simulink model "Problem1"  (R2020b)
settings: Solver=VariableStepAuto  StartTime=0.0  StopTime=100  MaxStep=0.01  RelTol=1e-3
model workspace (MAT data in the model file):
  K12 = 5000
  M2 = 50
undefined symbols (not defined in the file): b, K1, M1
settings Model: Creator=Hp  LastModifiedBy=Makrand Raut Dessai

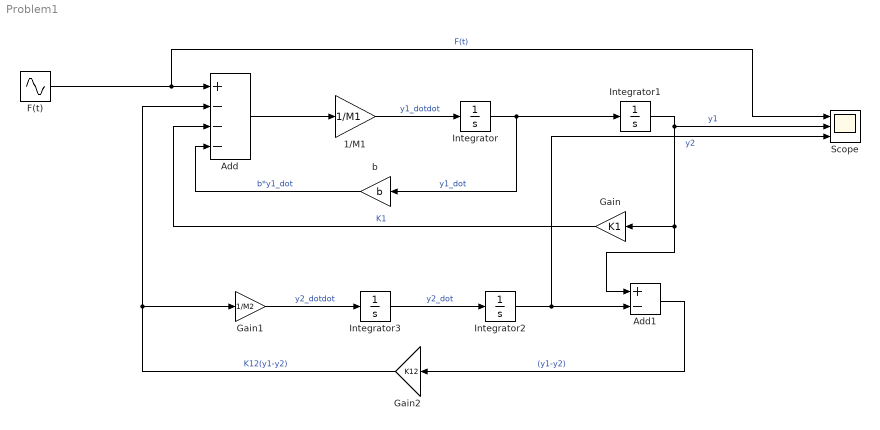
== system Problem1 ==
  1/M1 : Gain  Gain=1/M1
  Add : Sum  Inputs=+---
  Add1 : Sum  Inputs=+-
  F(t) : Sin  Amplitude=2  Frequency=10  SampleTime=0
  Gain : Gain  Gain=K1
  Gain1 : Gain  Gain=1/M2
  Gain2 : Gain  Gain=K12
  Integrator{,1..3} (4 alike) : Integrator
  Scope : Scope  NumInputPorts=3
  b : Gain  Gain=b
  wires:
  Gain2/1 -> Gain1/1, Add/2  "K12(y1-y2)"
  Add1/1 -> Gain2/1  "(y1-y2)"
  Integrator3/1 -> Integrator2/1  "y2_dot"
  1/M1/1 -> Integrator/1  "y1_dotdot"
  Integrator1/1 -> Scope/2, Gain/1, Add1/1  "y1"
  Gain/1 -> Add/3  "K1"
  Integrator/1 -> b/1, Integrator1/1  "y1_dot"
  Integrator2/1 -> Scope/3, Add1/2  "y2"
  Add/1 -> 1/M1/1
  b/1 -> Add/4  "b*y1_dot"
  Gain1/1 -> Integrator3/1  "y2_dotdot"
  F(t)/1 -> Scope/1, Add/1  "F(t)"
